simulink model "Test_Bed"  (R2020a)
settings: Solver=VariableStepAuto  StartTime=0.0  StopTime=10  FixedStep=10e-3  RelTol=1e-3
settings Model: Creator=LENOVO PC  LastModifiedBy=User Account

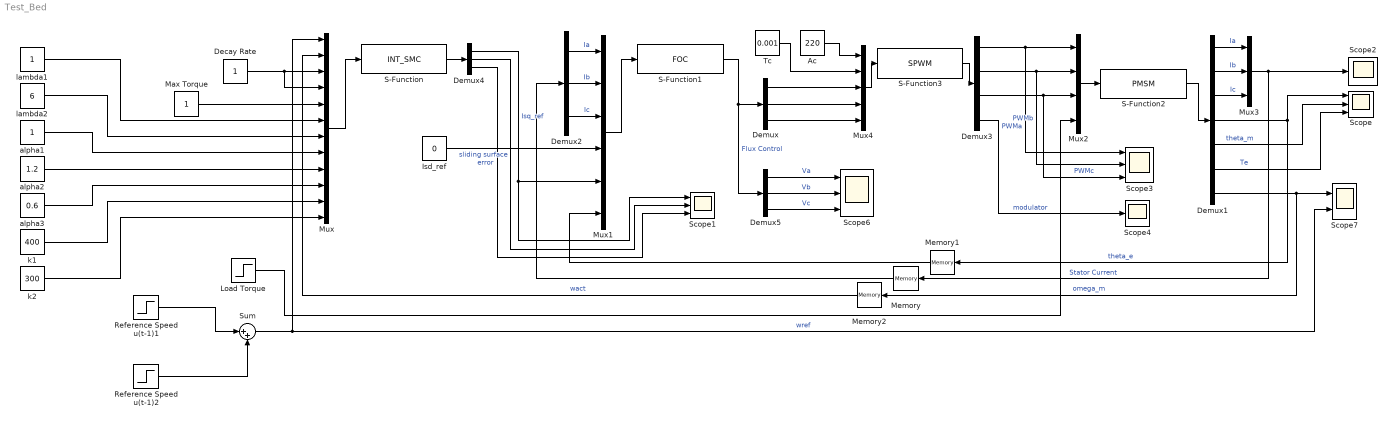
== system Test_Bed ==
  Ac : Constant  Value=220
  Decay Rate : Constant
  Demux{,2,4..5} (4 alike) : Demux  Outputs=3
  Demux1 : Demux  Outputs=7
  Demux3 : Demux
  Isd_ref : Constant  Value=0
  Load Torque : Step  Time=5  After=0  SampleTime=0
  Max Torque : Constant
  Memory : Memory
  Memory1 : Memory
  Memory2 : Memory
  Mux : Mux  Inputs=12
  Mux1 : Mux  Inputs=6
  Mux2 : Mux
  Mux3 : Mux  Inputs=3
  Mux4 : Mux  Inputs=5
  Reference Speed u(t-1)1 : Step  After=10  SampleTime=0
  Reference Speed u(t-1)2 : Step  Time=3  After=-5  SampleTime=0
  S-Function : S-Function  FunctionName=INT_SMC  SFunctionDeploymentMode=off  EnableBusSupport=off
  S-Function1 : S-Function  FunctionName=FOC  SFunctionDeploymentMode=off  EnableBusSupport=off
  S-Function2 : S-Function  FunctionName=PMSM  SFunctionDeploymentMode=off  EnableBusSupport=off
  S-Function3 : S-Function  FunctionName=SPWM  SFunctionDeploymentMode=off  EnableBusSupport=off
  Scope{,1,3,6} (4 alike) : Scope  NumInputPorts=3
  Scope2 : Scope
  Scope4 : Scope
  Scope7 : Scope  NumInputPorts=2
  Sum : Sum  Inputs=|++
  Tc : Constant  Value=0.001
  alpha1 : Constant
  alpha2 : Constant  Value=1.2
  alpha3 : Constant  Value=0.6
  k1 : Constant  Value=400
  k2 : Constant  Value=300
  lambda1 : Constant
  lambda2 : Constant  Value=6
  wires:
  Mux/1 -> S-Function/1
  Mux4/1 -> S-Function3/1
  Memory2/1 -> Mux/2  "wact"
  Memory/1 -> Demux2/1
  Mux2/1 -> S-Function2/1
  Demux1/3 -> Mux3/3  "Ic"
  Mux3/1 -> Scope2/1, Memory/1  "Stator Current"
  Demux1/2 -> Mux3/2  "Ib"
  S-Function2/1 -> Demux1/1
  Demux1/1 -> Mux3/1  "Ia"
  Load Torque/1 -> Mux2/4
  S-Function1/1 -> Demux5/1, Demux/1  "Flux Control"
  S-Function3/1 -> Demux3/1
  Mux1/1 -> S-Function1/1
  Demux1/4 -> Memory1/1, Scope/1  "theta_e"
  Demux1/5 -> Scope/2  "theta_m"
  Demux1/6 -> Scope/3  "Te"
  Demux1/7 -> Memory2/1, Scope7/1  "omega_m"
  Demux3/1 -> Mux2/1, Scope3/1  "PWMa"
  Demux3/2 -> Mux2/2, Scope3/2  "PWMb"
  Demux3/3 -> Mux2/3, Scope3/3  "PWMc"
  Demux3/4 -> Scope4/1  "modulator"
  Demux5/1 -> Scope6/1  "Va"
  Demux5/2 -> Scope6/2  "Vb"
  Demux5/3 -> Scope6/3  "Vc"
  S-Function/1 -> Demux4/1
  Reference Speed u(t-1)1/1 -> Sum/1
  Reference Speed u(t-1)2/1 -> Sum/2
  Sum/1 -> Scope7/2, Mux/1  "wref"
  Demux4/1 -> Mux1/5, Scope1/1  "Isq_ref"
  Demux4/2 -> Scope1/2  "sliding surface"
  Demux4/3 -> Scope1/3  "error"
  Decay Rate/1 -> Mux/4, Mux/3
  Max Torque/1 -> Mux/5
  lambda1/1 -> Mux/6
  lambda2/1 -> Mux/7
  alpha1/1 -> Mux/8
  alpha2/1 -> Mux/9
  alpha3/1 -> Mux/10
  k1/1 -> Mux/11
  k2/1 -> Mux/12
  Ac/1 -> Mux4/1
  Tc/1 -> Mux4/2
  Demux/1 -> Mux4/3
  Demux/2 -> Mux4/4
  Demux/3 -> Mux4/5
  Demux2/1 -> Mux1/1  "Ia"
  Demux2/2 -> Mux1/2  "Ib"
  Demux2/3 -> Mux1/3  "Ic"
  Isd_ref/1 -> Mux1/4
  Memory1/1 -> Mux1/6
